simulink model "daredevil_simulink"  (R2025b)
settings: Solver=VariableStepAuto  StartTime=0.0  StopTime=10.0  RelTol=1e-3
libraries: simulink x2
settings Model: Creator=ShwethaSharan T  LastModifiedBy=ShwethaSharan T

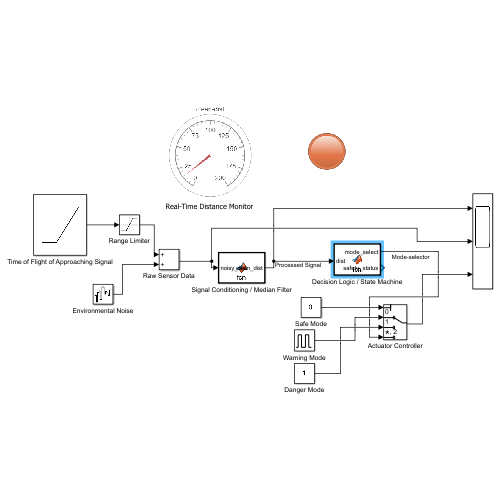
[thumbnail: Simulink's stored preview of the top-level diagram]
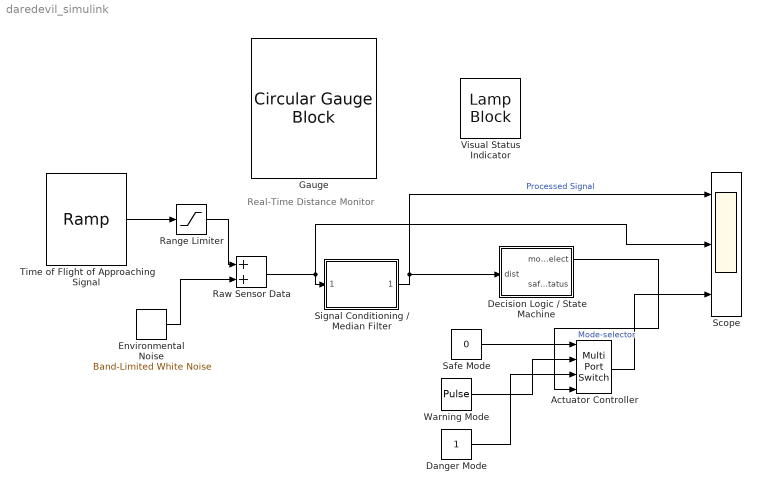
== system daredevil_simulink ==
  note: Real-Time Distance Monitor
  Actuator Controller : MultiPortSwitch  DataPortOrder=Zero-based contiguous  zeroidx=on  SaturateOnIntegerOverflow=off  InputSameDT=off
  Danger Mode : Constant
  Decision Logic / State Machine : MATLAB Function  TreatAsAtomicUnit=on
  Environmental Noise : simulink/Sources/Band-Limited White Noise  Cov=50  Ts=0.1  seed=[23341]
  Gauge : CircularGaugeBlock  ScaleMax=200  FontColor=[0.0, 0.0, 0.0]
  Range Limiter : Saturate  UpperLimit=250  LowerLimit=0
  Raw Sensor Data : Sum
  Safe Mode : Constant  Value=0
  Scope : Scope  NumInputPorts=3
      settings: ActiveDisplayYMinimum=-34.325711389790527  ActiveDisplayYMaximum=234.89396552591268
  Signal Conditioning / Median Filter : MATLAB Function  TreatAsAtomicUnit=on
  Time of Flight of Approaching Signal : simulink/Sources/Ramp  slope=-20  start=0  InitialOutput=200
  Visual Status Indicator : LampBlock  LabelPosition=Hide  DefaultColor=[192.0, 192.0, 192.0]
  Warning Mode : DiscretePulseGenerator  PulseType=Time based  Period=0.5  PulseWidth=50
  wires:
  Time of Flight of Approaching Signal/1 -> Range Limiter/1
  Range Limiter/1 -> Raw Sensor Data/1
  Environmental Noise/1 -> Raw Sensor Data/2
  Raw Sensor Data/1 -> Scope/2, Signal Conditioning / Median Filter/1(noisy_dist)
  Signal Conditioning / Median Filter/1(clean_dist) -> Scope/1, Decision Logic / State Machine/1(dist)  "Processed Signal"
  Decision Logic / State Machine/1(mode_select) -> Actuator Controller/4  "Mode-selector"
  Actuator Controller/1 -> Scope/3
  Safe Mode/1 -> Actuator Controller/1
  Warning Mode/1 -> Actuator Controller/2
  Danger Mode/1 -> Actuator Controller/3

== matlab function daredevil_simulink/Signal Conditioning // Median Filter ==
  data: noisy_dist input; clean_dist output
function clean_dist = fcn(noisy_dist)
    % Tactical Median Filter
    % Stores the last 5 samples to remove spikes
    persistent buffer
    if isempty(buffer)
        buffer = zeros(5,1);
    end

    % Shift buffer and add new value
    buffer(1:end-1) = buffer(2:end);
    buffer(end) = noisy_dist;

    % Calculate Median
    clean_dist = median(buffer);
end

== matlab function daredevil_simulink/Decision Logic // State Machine ==
  data: dist input; mode_select output; safety_status output
function [mode_select, safety_status] = fcn(dist)
    % Mode 0 = Safe (Off)
    % Mode 1 = Warning (Pulse)
    % Mode 2 = Danger (Solid)

    if dist > 120
        mode_select = 0; % Safe
        safety_status = 1; % Green Light
    elseif dist <= 120 && dist > 50
        mode_select = 1; % Warning Pulse
        safety_status = 0; % Yellow Light
    else
        mode_select = 2; % Critical Solid
        safety_status = -1; % Red Light
    end
end
